simulink model "Drone_sim"  (R2020a)
settings: Solver=FixedStepAuto  StartTime=0.0  StopTime=20  FixedStep=0.01  RelTol=1e-3
InitFcn:
  | Drone_Parameters;
values from neighbouring files (symbols this model uses):
  p0 = [0;0;0]    [Drone_Parameters.m]
  R0 = [cos(psi0) -sin(psi0) 0; sin(psi0) cos(psi0) 0; 0 0 1]    [Drone_Parameters.m]
settings Model: Creator=vcichella  LastModifiedBy=vcichella

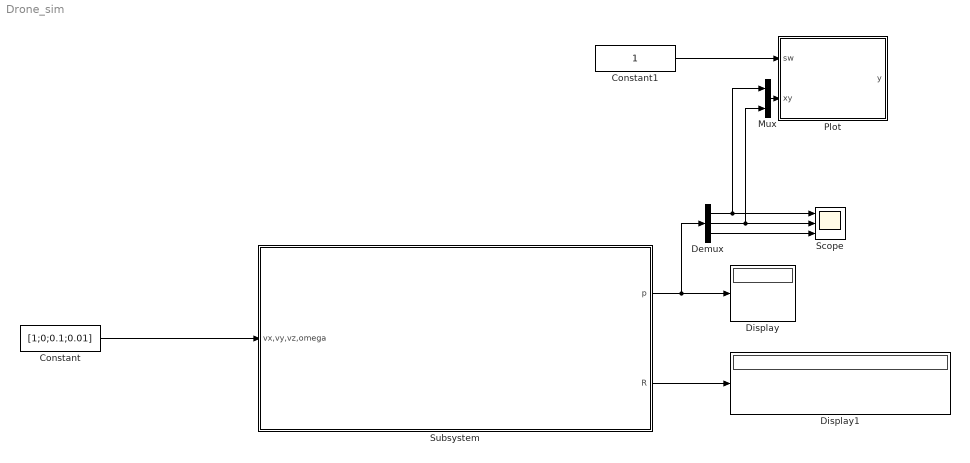
== system Drone_sim ==
  Constant : Constant  Value=[1;0;0.1;0.01]
  Constant1 : Constant
  Demux : Demux  Outputs=3
  Display : Display
  Display1 : Display
  Mux : Mux  Inputs=2
  Plot : MATLAB Function  TreatAsAtomicUnit=on
  Scope : Scope  NumInputPorts=3
  Subsystem : Subsystem
  wires:
  Constant/1 -> Subsystem/1(vx,vy,vz,omega)
  Subsystem/1(p) -> Demux/1, Display/1
  Subsystem/2(R) -> Display1/1
  Demux/1 -> Mux/1, Scope/1
  Demux/2 -> Mux/2, Scope/2
  Demux/3 -> Scope/3
  Constant1/1 -> Plot/1(sw)
  Mux/1 -> Plot/2(xy)

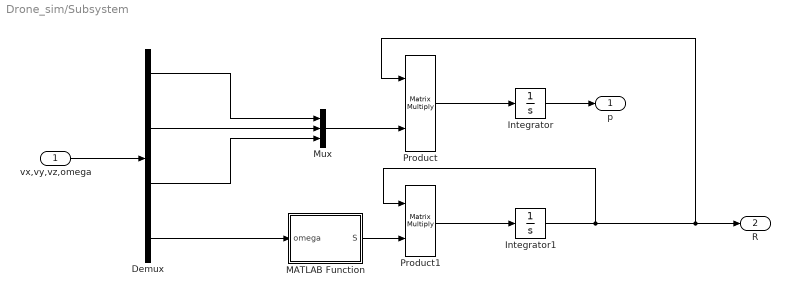
== system Drone_sim/Subsystem ==
  vx,vy,vz,omega : Inport
  Demux : Demux
  Integrator : Integrator  InitialCondition=p0
  Integrator1 : Integrator  InitialCondition=R0
  MATLAB Function : MATLAB Function  TreatAsAtomicUnit=on
  Mux : Mux  Inputs=3
  Product : Product  Multiplication=Matrix(*)
  Product1 : Product  Multiplication=Matrix(*)
  p : Outport
  R : Outport  Port=2
  wires:
  Integrator/1 -> p/1
  Integrator1/1 -> Product1/1, Product/1, R/1
  vx,vy,vz,omega/1 -> Demux/1
  Product/1 -> Integrator/1
  Mux/1 -> Product/2
  Demux/1 -> Mux/1
  Demux/2 -> Mux/2
  Demux/3 -> Mux/3
  Demux/4 -> MATLAB Function/1(omega)
  Product1/1 -> Integrator1/1
  MATLAB Function/1(S) -> Product1/2

== matlab function Drone_sim/Plot ==
  settings: updateMethod=DISCRETE
  settings: fimath=|
      | fimath(...
      | 'RoundMode', 'floor',...
      | 'OverflowMode', 'wrap',...
      | 'ProductMode', 'KeepLSB', 'ProductWordLength', 32,...
      | 'SumMode', 'KeepLSB', 'SumWordLength', 32,...
      | 'CastBeforeSum', false)
  data: sw input; xy input; y output
function y = plot3D(sw,xy)

persistent h k

eml.extrinsic('animatedline');
eml.extrinsic('addpoints');
eml.extrinsic('drawnow');
eml.extrinsic('clearpoints');

if isempty(k)
    k = 0;
end

if isempty(h)
   
    h = animatedline('Marker','d','Color','b'); hold on
    figure(1)
    hold on
    axis([-50 50 -50 50]);
%    axis equal
    grid on

end


addpoints(h,xy(1),xy(2));
drawnow
if sw > 1 & k == 0
    clearpoints(h);
    k = 1;
end

if sw == 0 
    k = 0;
end



y = 0;

== matlab function Drone_sim/Subsystem/MATLAB Function ==
  data: omega input; S output
function S = fcn(omega)

S = [0 -omega 0 ; omega 0 0; 0 0 0];
